simulink model "Velo_Complet_BF"  (R2018a)
settings: Solver=ode15s  StartTime=0.0  StopTime=5  FixedStep=0.0001  RelTol=1e-3
undefined symbols (not defined in the file): Kd_m, Kd_v, Ki_m, Ki_v, Kp_m, Kp_v
settings Model: Creator=chsira  LastModifiedBy=charl
settings DebuggingCC: LibraryContextMissingDiagnostic=warning
settings SFSimCC: SimUseLocalCustomCode=on
settings RTWCC: RTWUseLocalCustomCode=on

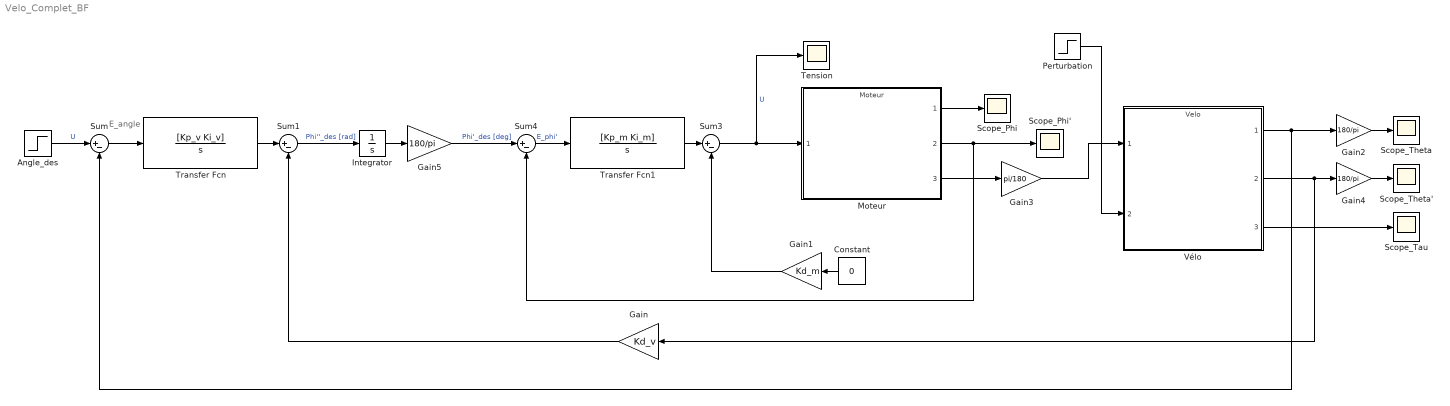
== system Velo_Complet_BF ==
  note: E_angle
  "Angle_des " : Step  Time=0  After=0  SampleTime=0
  Constant : Constant  Value=0
  Gain : Gain  Gain=Kd_v
  Gain1 : Gain  Gain=Kd_m
  Gain2 : Gain  Gain=180/pi
  Gain3 : Gain  Gain=pi/180
  Gain4 : Gain  Gain=180/pi
  Gain5 : Gain  Gain=180/pi
  Integrator : Integrator
  Moteur : ModelReference  ModelNameDialog=Moteur  SimulationMode=Normal  ModelReferenceVersion=1.29
  "Perturbation " : Step  Time=0  After=0  SampleTime=0
  Scope_Phi : Scope
  Scope_Phi' : Scope
  Scope_Tau : Scope
  Scope_Theta : Scope
  Scope_Theta' : Scope
  Sum{,1,3..4} (4 alike) : Sum  Inputs=|+-
  Tension : Scope
  Transfer Fcn : TransferFcn  Numerator=[Kp_v Ki_v]  Denominator=[1 0]
  Transfer Fcn1 : TransferFcn  Numerator=[Kp_m Ki_m]  Denominator=[1 0]
  Vélo : ModelReference  ModelNameDialog=Velo  ParameterArgumentNames=InitialCondition  ParameterArgumentValues=InitialCondition  UsingDefaultArgumentValue=0  SimulationMode=Normal  ModelReferenceVersion=1.66  InitialCondition=15*pi/180  SimulationMode=Normal
  wires:
  Moteur/1 -> Scope_Phi/1
  Vélo/2 -> Gain/1, Gain4/1
  Moteur/3 -> Gain3/1
  Vélo/3 -> Scope_Tau/1
  "Angle_des "/1 -> Sum/1  "U"
  Vélo/1 -> Sum/2, Gain2/1
  Sum/1 -> Transfer Fcn/1
  Transfer Fcn/1 -> Sum1/1
  Gain/1 -> Sum1/2
  Sum1/1 -> Integrator/1  "Phi''_des [rad]"
  Sum3/1 -> Tension/1, Moteur/1  "U"
  Transfer Fcn1/1 -> Sum3/1
  Gain1/1 -> Sum3/2
  Sum4/1 -> Transfer Fcn1/1  "E_phi'"
  Moteur/2 -> Scope_Phi'/1, Sum4/2
  Gain2/1 -> Scope_Theta/1
  Gain4/1 -> Scope_Theta'/1
  Integrator/1 -> Gain5/1
  "Perturbation "/1 -> Vélo/2
  Gain3/1 -> Vélo/1
  Gain5/1 -> Sum4/1  "Phi'_des [deg]"
  Constant/1 -> Gain1/1
